simulink model "model"  (R2022b)
settings: Solver=ode4  StartTime=0.0  StopTime=100  FixedStep=0.01  RelTol=1e-3
InitFcn:
  | load_data
values from neighbouring files (symbols this model uses):
  omega_n = 10    [extra.m]    (also in load_data.m; make_data.m)
  zeta = 0.3    [extra.m]    (also in load_data.m; make_data.m)
libraries: simulink x1
settings Model: Creator=Ali  LastModifiedBy=Ali

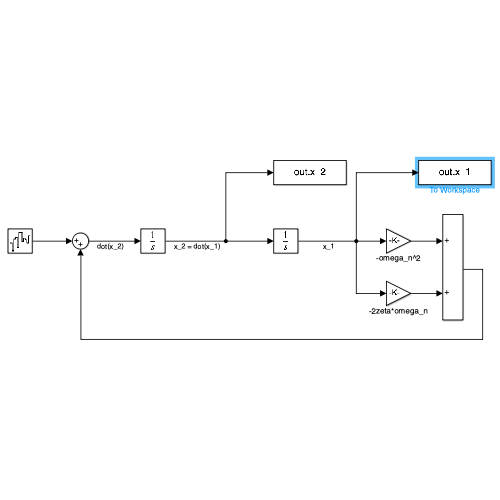
[thumbnail: Simulink's stored preview of the top-level diagram]
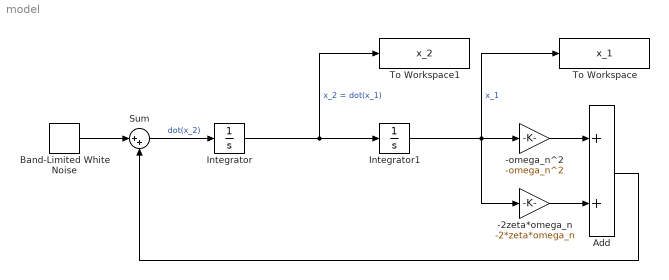
== system model ==
  -2zeta*omega_n : Gain  Gain=-2*zeta*omega_n
  -omega_n^2 : Gain  Gain=-omega_n^2
  Add : Sum
  Band-Limited White Noise : simulink/Sources/Band-Limited White Noise  Cov=1  Ts=0.01  seed=rand_seed
  Integrator : Integrator
  Integrator1 : Integrator
  Sum : Sum  Inputs=|++
  To Workspace : ToWorkspace  VariableName=x_1  SampleTime=-1
  To Workspace1 : ToWorkspace  VariableName=x_2  SampleTime=-1
  wires:
  Integrator/1 -> To Workspace1/1, Integrator1/1  "x_2 = dot(x_1)"
  Integrator1/1 -> To Workspace/1, -2zeta*omega_n/1, -omega_n^2/1  "x_1"
  Sum/1 -> Integrator/1  "dot(x_2)"
  -2zeta*omega_n/1 -> Add/2
  -omega_n^2/1 -> Add/1
  Add/1 -> Sum/2
  Band-Limited White Noise/1 -> Sum/1
